simulink model "ochoPSKImageTransfer_Comprimida_ConMultiplexacion_Completado"  (R2016a)
settings: Solver=VariableStepDiscrete  SolverMode=SingleTasking  StartTime=0.0  StopTime=420800  RelTol=1e-3
libraries: commlibv2 x8, commutil2 x6, commdigbbndpm3 x6, commchan3 x1, commhdledac x1, commhdllib x1, commdigbbnd2 x1
settings Model: Creator=Glynis  LastModifiedBy=Glynis
settings DataIOCC: LimitDataPoints=on  SaveOutput=off  SaveTime=off
settings OptimizationCC: BooleanDataType=off  DefaultParameterBehavior=Inlined  LocalBlockOutputs=off
settings DebuggingCC: AlgebraicLoopMsg=error  SingleTaskRateTransMsg=error  AllowSymbolicDim=off
settings ConfigComp: CovModelRefEnable=Off  CovSFcnEnable=off

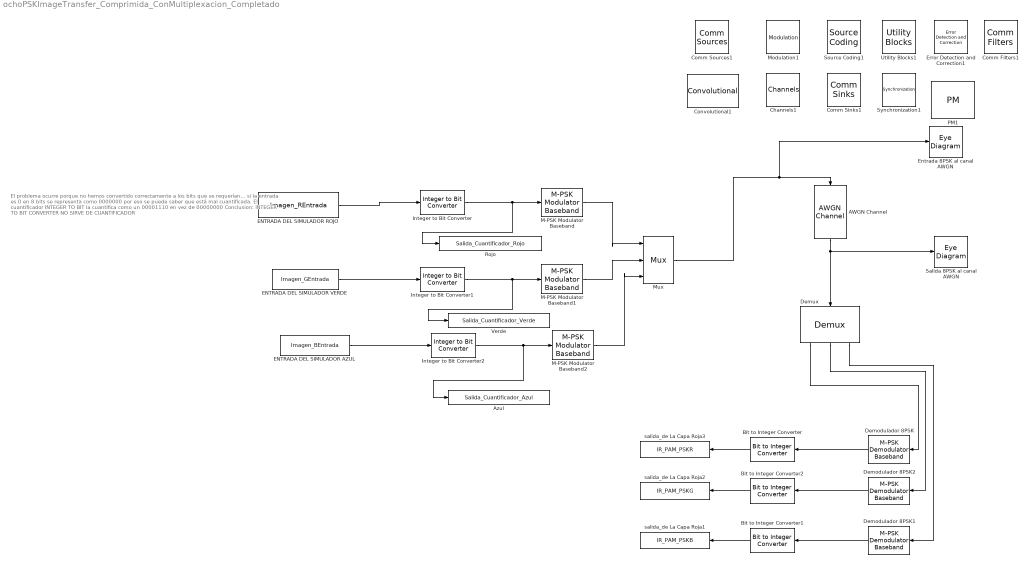
== system ochoPSKImageTransfer_Comprimida_ConMultiplexacion_Completado ==
  note: El problema ocurre porque no hemos convertido correctamente a los bits que se requerían...
      | si la entrada es 0 en 8 bits se representa como 0000000 por eso se puede saber que
      | está mal cuantificada.
      |
      | El cuantificador INTEGER TO BIT la cuantifica como un
      | 00001110
      | en vez de
      | 00000000
      |
      | Conclusion: INTEGER TO BIT CONVERTER NO SIRVE DE CUANTIFICADOR
  AWGN Channel : commchan3/AWGN Channel  InputProcessing=Columns as channels (frame based)  seed=654  noiseMode="Signal to noise ratio  (Eb/No)"  EbNodB=100  EsNodB=10  SNRdB=10  bitsPerSym=8  Ps=1000  Tsym=1  variance=1
  Azul : ToWorkspace  VariableName=Salida_Cuantificador_Azul  SampleTime=-1
      settings: Save2DSignal=2-D array (concatenate along first dimension)
  Bit to Integer Converter : commutil2/Bit to Integer Converter  nbits=8  bitOrder=MSB first  signedOutputValues=Unsigned  outDtype=double  outDtypeSigned=Inherit via internal rule
  Bit to Integer Converter1 : commutil2/Bit to Integer Converter  nbits=8  bitOrder=MSB first  signedOutputValues=Unsigned  outDtype=double  outDtypeSigned=Inherit via internal rule
  Bit to Integer Converter2 : commutil2/Bit to Integer Converter  nbits=8  bitOrder=MSB first  signedOutputValues=Unsigned  outDtype=double  outDtypeSigned=Inherit via internal rule
  Channels1 : commlibv2/Channels
  Comm Filters1 : commlibv2/Comm Filters
  Comm Sinks1 : commlibv2/Comm Sinks
  Comm Sources1 : commlibv2/Comm Sources
  Convolutional1 : commhdledac/Convolutional
  Demodulador 8PSK : commdigbbndpm3/M-PSK Demodulator Baseband  M=8  OutType=Integer  DecType=Hard decision  VarSource=Dialog  Variance=1  Dec=Gray  Mapping=[0:7]  Ph=pi/8  outDtype1=Inherit via internal rule  outDtype2=Inherit via internal rule  derotateFactorWordLen=16  derotateFactorDataTypeStr=Inherit: Same word length as input  derotateFactorLastDataTypeStr=Inherit: Same word length as input
  Demodulador 8PSK1 : commdigbbndpm3/M-PSK Demodulator Baseband  M=8  OutType=Integer  DecType=Hard decision  VarSource=Dialog  Variance=1  Dec=Gray  Mapping=[0:7]  Ph=pi/8  outDtype1=Inherit via internal rule  outDtype2=Inherit via internal rule  derotateFactorWordLen=16  derotateFactorDataTypeStr=Inherit: Same word length as input  derotateFactorLastDataTypeStr=Inherit: Same word length as input
  Demodulador 8PSK2 : commdigbbndpm3/M-PSK Demodulator Baseband  M=8  OutType=Integer  DecType=Hard decision  VarSource=Dialog  Variance=1  Dec=Gray  Mapping=[0:7]  Ph=pi/8  outDtype1=Inherit via internal rule  outDtype2=Inherit via internal rule  derotateFactorWordLen=16  derotateFactorDataTypeStr=Inherit: Same word length as input  derotateFactorLastDataTypeStr=Inherit: Same word length as input
  Demux : Demux  Outputs=3
  ENTRADA DEL SIMULADOR AZUL : FromWorkspace  VariableName=Imagen_BEntrada  SampleTime=1  OutputAfterFinalValue=Holding final value
  ENTRADA DEL SIMULADOR ROJO : FromWorkspace  VariableName=Imagen_REntrada  SampleTime=1  OutputAfterFinalValue=Holding final value
  ENTRADA DEL SIMULADOR VERDE : FromWorkspace  VariableName=Imagen_GEntrada  SampleTime=1  OutputAfterFinalValue=Holding final value
  Entrada 8PSK al canal AWGN : EyeDiagram
  Error Detection and Correction1 : commhdllib/Error Detection and Correction
  Integer to Bit Converter : commutil2/Integer to Bit Converter  nbits=8  signedInputValues=Unsigned  bitOrder=MSB first  outDtype=double
  Integer to Bit Converter1 : commutil2/Integer to Bit Converter  nbits=8  signedInputValues=Unsigned  bitOrder=MSB first  outDtype=double
  Integer to Bit Converter2 : commutil2/Integer to Bit Converter  nbits=8  signedInputValues=Unsigned  bitOrder=MSB first  outDtype=double
  M-PSK Modulator Baseband : commdigbbndpm3/M-PSK Modulator Baseband  M=8  InType=Integer  Enc=Gray  Mapping=[0:7]  Ph=pi/8  outDtype=double  outWordLen=16  outUDDataType=sfix(16)  outFracLenMode=Best precision  outFracLen=15  outDataTypeStr=double  outLastDataTypeStr=double
  M-PSK Modulator Baseband1 : commdigbbndpm3/M-PSK Modulator Baseband  M=8  InType=Integer  Enc=Gray  Mapping=[0:7]  Ph=pi/8  outDtype=double  outWordLen=16  outUDDataType=sfix(16)  outFracLenMode=Best precision  outFracLen=15  outDataTypeStr=double  outLastDataTypeStr=double
  M-PSK Modulator Baseband2 : commdigbbndpm3/M-PSK Modulator Baseband  M=8  InType=Integer  Enc=Gray  Mapping=[0:7]  Ph=pi/8  outDtype=double  outWordLen=16  outUDDataType=sfix(16)  outFracLenMode=Best precision  outFracLen=15  outDataTypeStr=double  outLastDataTypeStr=double
  Modulation1 : commlibv2/Modulation
  Mux : Mux  Inputs=3
      settings: DisplayOption=signals
  PM1 : commdigbbnd2/PM
  Rojo : ToWorkspace  VariableName=Salida_Cuantificador_Rojo  SampleTime=-1
      settings: Save2DSignal=2-D array (concatenate along first dimension)
  Salida 8PSK al canal AWGN : EyeDiagram
  Source Coding1 : commlibv2/Source Coding
  Synchronization1 : commlibv2/Synchronization
  Utility Blocks1 : commlibv2/Utility Blocks
  "Verde " : ToWorkspace  VariableName=Salida_Cuantificador_Verde  SampleTime=-1
      settings: Save2DSignal=2-D array (concatenate along first dimension)
  salida_de La Capa Roja1 : ToWorkspace  VariableName=IR_PAM_PSKB  SampleTime=1
      settings: Save2DSignal=2-D array (concatenate along first dimension)
  salida_de La Capa Roja2 : ToWorkspace  VariableName=IR_PAM_PSKG  SampleTime=1
      settings: Save2DSignal=2-D array (concatenate along first dimension)
  salida_de La Capa Roja3 : ToWorkspace  VariableName=IR_PAM_PSKR  SampleTime=1
      settings: Save2DSignal=2-D array (concatenate along first dimension)
  wires:
  Integer to Bit Converter/1 -> M-PSK Modulator Baseband/1, Rojo/1
  Bit to Integer Converter/1 -> salida_de La Capa Roja3/1
  ENTRADA DEL SIMULADOR ROJO/1 -> Integer to Bit Converter/1
  Demodulador 8PSK/1 -> Bit to Integer Converter/1
  AWGN Channel/1 -> Demux/1, Salida 8PSK al canal AWGN/1
  Mux/1 -> Entrada 8PSK al canal AWGN/1, AWGN Channel/1
  Demux/1 -> Demodulador 8PSK/1
  Bit to Integer Converter1/1 -> salida_de La Capa Roja1/1
  Demodulador 8PSK1/1 -> Bit to Integer Converter1/1
  Bit to Integer Converter2/1 -> salida_de La Capa Roja2/1
  Demodulador 8PSK2/1 -> Bit to Integer Converter2/1
  Demux/2 -> Demodulador 8PSK2/1
  Demux/3 -> Demodulador 8PSK1/1
  M-PSK Modulator Baseband/1 -> Mux/1
  Integer to Bit Converter1/1 -> M-PSK Modulator Baseband1/1, "Verde "/1
  ENTRADA DEL SIMULADOR VERDE/1 -> Integer to Bit Converter1/1
  M-PSK Modulator Baseband1/1 -> Mux/2
  Integer to Bit Converter2/1 -> M-PSK Modulator Baseband2/1, Azul/1
  ENTRADA DEL SIMULADOR AZUL/1 -> Integer to Bit Converter2/1
  M-PSK Modulator Baseband2/1 -> Mux/3
